simulink model "MicrogridControl"  (R2025b)
settings: Solver=VariableStepAuto  StartTime=0.0  StopTime=8  FixedStep=Ts  RelTol=1e-3
PreLoadFcn:
  | NormalOperation;
  | MicrogridControlParam;
undefined symbols (not defined in the file): base, bessModeInitial, bessSystem, bessVoltage, breakerStatus, DiscIntNeverNeededParam, ee_sli_rtmsupport, event, gcbh, generator, gflInverter, gfmInverter, Inertia, lineInductance, lineResistance, machine, plannedIsland, pmsm, powerLimit, powerQuality, PV, PVInverter, ref, resync, solar, solarInsolationChange, systemFrequency, Ts, windController, windSystem, windTurbine
libraries: nesl_utility x234, ee_lib x174, fl_lib x143, eeGeneralControl x137, simulink x78, eeTransforms x47, slpidlib x23, nesl_utility_internal x12, eePwmGenerator x9, eeSinusoidalMeasurementV2 x9, custom_lib x7, batteryecm_lib x6
(part 20 of 25)

== system MicrogridControl/BESS/BESS Integrated/Detailed/BESS Controller/Grid Forming/Power Control/ReactiveControl/Voltage  Reference Selection ==
  cntrlflag : Inport
  Qref : Inport  Port=2
  Qmeas : Inport  Port=3
  Vref : Inport  Port=4
  Vgdmeas : Inport  Port=5
  If : If
  If Action Subsystem : Subsystem  TreatAsAtomicUnit=on
  If Action Subsystem1 : Subsystem  TreatAsAtomicUnit=on
  Merge : Merge
  Rate Transition : RateTransition
  Vd : Outport
  wires:
  Rate Transition/1 -> If/1
  Vgdmeas/1 -> If Action Subsystem1/2(Vmeas)
  Vref/1 -> If Action Subsystem1/1(Vref)
  If Action Subsystem1/1(Voltage) -> Merge/2
  Qref/1 -> If Action Subsystem/1(Qref)
  Qmeas/1 -> If Action Subsystem/2(Qmeas)
  Merge/1 -> Vd/1
  cntrlflag/1 -> Rate Transition/1
  If/2 -> If Action Subsystem1/Action
  If Action Subsystem/1(Vd) -> Merge/1
  If/1 -> If Action Subsystem/Action

== system MicrogridControl/BESS/BESS Integrated/Detailed/BESS Controller/Grid Forming/VoltageCurrentControl/Controller/Id Current Limiting ==
  Imax : Inport
  Id : Inport  Port=2
  Abs : Abs  SaturateOnIntegerOverflow=off
  Switch : Switch  Criteria=u2 > Threshold  SaturateOnIntegerOverflow=off  InputSameDT=off
  Idref : Outport
  wires:
  Switch/1 -> Idref/1
  Imax/1 -> Switch/1, Abs/1
  Abs/1 -> Switch/2
  Id/1 -> Switch/3

== system MicrogridControl/BESS/BESS Integrated/Detailed/BESS Controller/Grid Forming/VoltageCurrentControl/Controller/Iq Current Limiting ==
  Imax : Inport
  Iq : Inport  Port=2
  Abs : Abs  SaturateOnIntegerOverflow=off
  Switch : Switch  Criteria=u2 > Threshold  SaturateOnIntegerOverflow=off  InputSameDT=off
  Iqref : Outport
  wires:
  Switch/1 -> Iqref/1
  Imax/1 -> Switch/1, Abs/1
  Abs/1 -> Switch/2
  Iq/1 -> Switch/3

== system MicrogridControl/BESS/BESS Integrated/Detailed/BESS Controller/Grid Forming/VoltageCurrentControl/Controller/Voltage control ==
  e : Inport
  resetBlackStart : Inport  Port=2
  Discrete-Time Integrator : DiscreteIntegrator  IntegratorMethod=Integration: Backward Euler  ExternalReset=level  SampleTime=voltControlTs  LimitOutput=on  UpperSaturationLimit=VdMaxCt  LowerSaturationLimit=VdMinCt  ICPrevOutput=DiscIntNeverNeededParam  ICPrevScaledInput=DiscIntNeverNeededParam
  Ki : Gain  Gain=VdIGain
  Kp : Gain  Gain=vdPGain
  Limit : Saturate  UpperLimit=VdMaxCt  LowerLimit=VdMinCt
  Scope : Scope  NumInputPorts=2
      settings: ActiveDisplayYMinimum=-2.29888  ActiveDisplayYMaximum=11.36654  DataLoggingVariableName=ScopeData7
  Scope1 : Scope
      settings: ActiveDisplayYMinimum=-0.22989  ActiveDisplayYMaximum=1.13665  DataLoggingVariableName=ScopeData8
  Sum7 : Sum  Inputs=|++
  u : Outport  VectorParamsAs1DForOutWhenUnconnected=off
  wires:
  resetBlackStart/1 -> Discrete-Time Integrator/2
  e/1 -> Scope1/1, Ki/1, Kp/1
  Sum7/1 -> Limit/1
  Ki/1 -> Discrete-Time Integrator/1
  Limit/1 -> u/1
  Kp/1 -> Scope/1, Sum7/1
  Discrete-Time Integrator/1 -> Scope/2, Sum7/2

== system MicrogridControl/BESS/BESS Integrated/Detailed/BESS Controller/Grid Forming/VoltageCurrentControl/Controller/Voltage control1 ==
  e : Inport
  resetBlackStart : Inport  Port=2
  Discrete-Time Integrator : DiscreteIntegrator  IntegratorMethod=Integration: Backward Euler  ExternalReset=level  SampleTime=voltControlTs  LimitOutput=on  UpperSaturationLimit=VqMaxCt  LowerSaturationLimit=VqMinCt  ICPrevOutput=DiscIntNeverNeededParam  ICPrevScaledInput=DiscIntNeverNeededParam
  Ki : Gain  Gain=VqIGain
  Kp : Gain  Gain=VqPGain
  Limit : Saturate  UpperLimit=VqMaxCt  LowerLimit=VqMinCt
  Sum7 : Sum  Inputs=|++
  u : Outport  VectorParamsAs1DForOutWhenUnconnected=off
  wires:
  resetBlackStart/1 -> Discrete-Time Integrator/2
  Limit/1 -> u/1
  Ki/1 -> Discrete-Time Integrator/1
  Kp/1 -> Sum7/1
  e/1 -> Kp/1, Ki/1
  Sum7/1 -> Limit/1
  Discrete-Time Integrator/1 -> Sum7/2

== system MicrogridControl/BESS/BESS Integrated/Detailed/BESS Controller/Grid Forming/VoltageCurrentControl/Controller/d-axis current control ==
  e : Inport
  resetBlackStart : Inport  Port=2
  Discrete-Time Integrator : DiscreteIntegrator  IntegratorMethod=Integration: Backward Euler  ExternalReset=level  SampleTime=currentControlTs  LimitOutput=on  UpperSaturationLimit=4  LowerSaturationLimit=-4  ICPrevOutput=DiscIntNeverNeededParam  ICPrevScaledInput=DiscIntNeverNeededParam
  Ki : Gain  Gain=IdIGain
  Kp : Gain  Gain=IdPGain
  Limit : Saturate  UpperLimit=4  LowerLimit=-4
  Sum7 : Sum  Inputs=|++
  u : Outport  VectorParamsAs1DForOutWhenUnconnected=off
  wires:
  resetBlackStart/1 -> Discrete-Time Integrator/2
  Ki/1 -> Discrete-Time Integrator/1
  Limit/1 -> u/1
  Kp/1 -> Sum7/1
  e/1 -> Kp/1, Ki/1
  Sum7/1 -> Limit/1
  Discrete-Time Integrator/1 -> Sum7/2

== system MicrogridControl/BESS/BESS Integrated/Detailed/BESS Controller/Grid Forming/VoltageCurrentControl/Controller/q-axis current control ==
  e : Inport
  resetBlackStart : Inport  Port=2
  Discrete-Time Integrator : DiscreteIntegrator  IntegratorMethod=Integration: Backward Euler  ExternalReset=level  SampleTime=currentControlTs  LimitOutput=on  UpperSaturationLimit=3  LowerSaturationLimit=-3  ICPrevOutput=DiscIntNeverNeededParam  ICPrevScaledInput=DiscIntNeverNeededParam
  Ki : Gain  Gain=IqIGain
  Kp : Gain  Gain=IqPGain
  Limit : Saturate  UpperLimit=3  LowerLimit=-3
  Sum7 : Sum  Inputs=|++
  u : Outport  VectorParamsAs1DForOutWhenUnconnected=off
  wires:
  resetBlackStart/1 -> Discrete-Time Integrator/2
  Discrete-Time Integrator/1 -> Sum7/2
  Limit/1 -> u/1
  Sum7/1 -> Limit/1
  e/1 -> Ki/1, Kp/1
  Kp/1 -> Sum7/1
  Ki/1 -> Discrete-Time Integrator/1

== system MicrogridControl/BESS/BESS Integrated1/Detailed/BESS Controller/Grid Forming/Current Limiting/CurrentLimitingMethod/currentLimitAndVirtual ==
  Igd : Inport
  Igq : Inport  Port=2
  Current Saturation : Subsystem
  CurrentLimitSelection : Stateflow chart  TreatAsAtomicUnit=on
  Math Function : Math  Operator=hypot
  Merge{,1..3} (4 alike) : Merge  Inputs=3
  No Fault Ride Through : Subsystem
  VI : Subsystem
  delVd : Outport
  delVq : Outport  Port=2
  Idmax : Outport  Port=3
  Iqmax : Outport  Port=4
  wires:
  [Imax] -> VI/3(Imax)
  [Imax] -> Current Saturation/3(Imaxsat)
  [noCtLt] -> No Fault Ride Through/Enable
  [satCtLt] -> Current Saturation/Enable
  [viCtLt] -> VI/Enable
  CurrentLimitSelection/4(satCurrentLimit) -> [satCtLt]
  CurrentLimitSelection/3(viCurrentLimit) -> [viCtLt]
  CurrentLimitSelection/2(noCurrentLimit) -> [noCtLt]
  CurrentLimitSelection/1(ismax) -> [Imax]
  Math Function/1 -> CurrentLimitSelection/1(Is)
  No Fault Ride Through/2(delVq) -> Merge1/3
  Merge3/1 -> Iqmax/1
  Current Saturation/2(delVq) -> Merge1/2
  No Fault Ride Through/4(iqmax) -> Merge3/3
  VI/3(idmax) -> Merge2/1
  VI/4(iqmax) -> Merge3/1
  Current Saturation/3(idmax) -> Merge2/2
  VI/2(delVq) -> Merge1/1
  Merge/1 -> delVd/1
  Current Saturation/4(iqmax) -> Merge3/2
  Current Saturation/1(delVd) -> Merge/2
  [Id] -> Math Function/1
  [Iq] -> Math Function/2
  VI/1(delVd) -> Merge/1
  No Fault Ride Through/3(idmax) -> Merge2/3
  No Fault Ride Through/1(delVd) -> Merge/3
  Igd/1 -> [Id], No Fault Ride Through/1(Id), Current Saturation/1(Id), VI/1(Id)
  Merge1/1 -> delVq/1
  Igq/1 -> [Iq], No Fault Ride Through/2(Iq), VI/2(Iq), Current Saturation/2(Iq)
  Merge2/1 -> Idmax/1

== system MicrogridControl/BESS/BESS Integrated1/Detailed/BESS Controller/Grid Forming/Current Limiting/CurrentLimitingMethod/currentSaturation ==
  note: Vs-delV
  Igd : Inport
  Igq : Inport  Port=2
  Compare : Subsystem
  Constant : Constant  Value=maxSatCurrentLimit
  Constant1 : Constant  Value=0
  Constant2 : Constant  Value=0
  If : If
  If Action Subsystem : Subsystem  TreatAsAtomicUnit=on
  If Action Subsystem1 : Subsystem  TreatAsAtomicUnit=on
  Math Function : Math  Operator=hypot
  Merge : Merge
  Merge1 : Merge
  Subtract : Sum  Inputs=+-
  delVd : Outport
  delVq : Outport  Port=2
  Idmax : Outport  Port=3
  Iqmax : Outport  Port=4
  wires:
  Merge1/1 -> Iqmax/1
  Merge/1 -> Idmax/1
  Constant1/1 -> delVd/1
  Constant2/1 -> delVq/1
  If Action Subsystem1/2(Iqmax) -> Merge1/2
  If Action Subsystem/2(Iqmax) -> Merge1/1
  If Action Subsystem1/1(Idmax) -> Merge/2
  If Action Subsystem/1(Idmax) -> Merge/1
  [Is] -> If Action Subsystem/1(Is)
  If/2 -> If Action Subsystem1/Action
  Compare/1(Out1) -> If/1
  Subtract/1 -> Compare/1(u)
  [Isq] -> If Action Subsystem/3(Isq)
  [Isd] -> If Action Subsystem/2(Isd)
  If/1 -> If Action Subsystem/Action
  Math Function/1 -> Subtract/2, [Is]  "Is"
  Constant/1 -> Subtract/1
  Igq/1 -> Math Function/2, [Isq]
  Igd/1 -> Math Function/1, [Isd]

== system MicrogridControl/BESS/BESS Integrated1/Detailed/BESS Controller/Grid Forming/Current Limiting/CurrentLimitingMethod/virtualImpedance ==
  note: Resistance coefficient
  note: X/R ratio
  Igd : Inport
  Igq : Inport  Port=2
  Constant : Constant  Value=maxVICurrentLimit
  Constant1 : Constant  Value=0
  Constant2 : Constant  Value=0
  Constant3 : Constant  Value=0
  Gain : Gain  Gain=ctLimitVirtualImp
  Gain1 : Gain  Gain=ctLimitXbyR
  Low-Pass Filter : eeGeneralControl/Low-Pass Filter (Discrete or Continuous)  K=1  T=currentVITimeConst  B=inf  A=-inf  init_option=Inherited from block input  x0=0  Ts=-1
  Math Function : Math  Operator=hypot
  Product{,1..3} (4 alike) : Product
  Relay : Relay  OnSwitchValue=0.01  OffSwitchValue=-0.05
  Saturation : Saturate  UpperLimit=1  LowerLimit=-1
  Saturation1 : Saturate  UpperLimit=1  LowerLimit=-1
  Sum : Sum  Inputs=|+-
  Sum1 : Sum  Inputs=|+-
  Sum2 : Sum  Inputs=++|
  Switch : Switch  Criteria=u2 > Threshold  SaturateOnIntegerOverflow=off  InputSameDT=off
  delVd : Outport
  delVq : Outport  Port=2
  Idmax : Outport  Port=3
  Iqmax : Outport  Port=4
  wires:
  Sum2/1 -> Saturation1/1
  Product3/1 -> Sum2/2
  Low-Pass Filter/1 -> Sum/1
  Saturation/1 -> delVd/1
  Relay/1 -> Switch/2
  Saturation1/1 -> delVq/1
  Igd/1 -> [Igd], Math Function/1
  Constant1/1 -> Switch/3
  Gain/1 -> Switch/1
  Constant3/1 -> Iqmax/1
  Constant2/1 -> Idmax/1
  [Igd] -> Product/2, Product1/1
  Switch/1 -> Product/1, Product3/2, Gain1/1
  [Igq] -> Product2/2, Product3/1
  Math Function/1 -> Low-Pass Filter/1  "Is"
  Constant/1 -> Sum/2  "IsMaxium"
  Product2/1 -> Sum1/2
  Product/1 -> Sum1/1
  Sum1/1 -> Saturation/1
  Gain1/1 -> Product2/1, Product1/2
  Product1/1 -> Sum2/1
  Igq/1 -> Math Function/2, [Igq]
  Sum/1 -> Relay/1, Gain/1

== system MicrogridControl/BESS/BESS Integrated1/Detailed/BESS Controller/Grid Forming/Grid Voltage Reactive Power Support/Modifying Active Power Reference/Computing New Active Power Ref ==
  Iq : Inport
  Vd : Inport  Port=2
  Abs : Abs  SaturateOnIntegerOverflow=off
  Constant : Constant  Value=maxVICurrentLimit*0.96
  Constant1 : Constant  Value=0
  Product : Product
  Sqrt : Sqrt
  Square : Math  Operator=square
  Square1 : Math  Operator=square
  Subtract : Sum  Inputs=-+
  Switch : Switch  Criteria=u2 > Threshold  Threshold=1.15  SaturateOnIntegerOverflow=off  InputSameDT=off
  Pref : Outport
  wires:
  Product/1 -> Pref/1
  Iq/1 -> Square/1
  Sqrt/1 -> Abs/1
  Vd/1 -> Product/1
  Constant1/1 -> Switch/1
  Square1/1 -> Subtract/2
  Square/1 -> Switch/2, Subtract/1
  Switch/1 -> Product/2
  Subtract/1 -> Sqrt/1
  Constant/1 -> Square1/1
  Abs/1 -> Switch/3

== system MicrogridControl/BESS/BESS Integrated1/Detailed/BESS Controller/Grid Forming/Grid Voltage Reactive Power Support/Modifying Reactive Power Reference/Changing the Power Reference ==
  Vs : Inport
  Vd : Inport  Port=2
  Pref : Inport  Port=3
  Qref : Inport  Port=4
  Enable : EnablePort
  ActivePowerReference : Subsystem
  Constant1 : Constant  Value=voltreference*0.96
  EstimateIdForGivenIq : Subsystem
  EstimateIqForReactivePower : Subsystem
  Max : MinMax  Function=max  Inputs=2
  ReactivePowerReference : Subsystem
  Prefv : Outport
  Qrefv : Outport  Port=2
  wires:
  Vd/1 -> EstimateIqForReactivePower/2(Vd)
  Qref/1 -> Max/2
  ReactivePowerReference/1(QrefNew) -> Max/1
  Pref/1 -> ActivePowerReference/3(Pref)
  EstimateIdForGivenIq/1(Id) -> ActivePowerReference/1(Id)
  Vs/1 -> ReactivePowerReference/1(Vd), EstimateIqForReactivePower/3(Vs), ActivePowerReference/2(Vd)
  Constant1/1 -> EstimateIqForReactivePower/1(Vmin)
  EstimateIqForReactivePower/1(Iq) -> ReactivePowerReference/2(Iq), EstimateIdForGivenIq/1(Iq)
  Max/1 -> Qrefv/1
  ActivePowerReference/1(PrefNew) -> Prefv/1

== system MicrogridControl/BESS/BESS Integrated1/Detailed/BESS Controller/Grid Forming/Grid Voltage Reactive Power Support/Modifying Reactive Power Reference/Hysteresis ==
  Vs : Inport
  AND : Logic  IconShape=distinctive  AllPortsSameDT=off  OutDataTypeStr=boolean
  Compare To Constant : simulink/Logic and Bit Operations/Compare To Constant  relop=<  const=0.9  OutDataTypeStr=boolean
  Compare To Constant1 : simulink/Logic and Bit Operations/Compare To Constant  relop=<  const=0.95  OutDataTypeStr=boolean
  D Latch : simulink_extras/Flip Flops/D Latch
  OR : Logic  Operator=OR  IconShape=distinctive  AllPortsSameDT=off  OutDataTypeStr=boolean
  Scope : Scope
      settings: ActiveDisplayYMinimum=0.96929  ActiveDisplayYMaximum=1.01111
  Terminator : Terminator
  LVFlag : Outport
  wires:
  Vs/1 -> Compare To Constant/1, Compare To Constant1/1, Scope/1
  Compare To Constant/1 -> OR/2, D Latch/2, D Latch/1
  D Latch/2 -> Terminator/1
  OR/1 -> LVFlag/1
  AND/1 -> OR/1
  D Latch/1 -> AND/2
  Compare To Constant1/1 -> AND/1

== system MicrogridControl/BESS/BESS Integrated1/Detailed/BESS Controller/Grid Forming/Grid Voltage Reactive Power Support/Modifying Reactive Power Reference/Not Altering the Power Reference ==
  Pref : Inport
  Qref : Inport  Port=2
  Enable : EnablePort
  Prefv : Outport
  Qrefv : Outport  Port=2
  wires:
  Qref/1 -> Qrefv/1
  Pref/1 -> Prefv/1

== system MicrogridControl/BESS/BESS Integrated1/Detailed/BESS Controller/Grid Forming/Measurement/Frequency Measurement/Frequency Measurement ==
  abc : Inport
  Constant : Constant
  Discrete-Time Integrator : DiscreteIntegrator  SampleTime=sampleTime  LimitOutput=on  ICPrevOutput=DiscIntNeverNeededParam  ICPrevScaledInput=DiscIntNeverNeededParam
  If : If  IfExpression=u1 > 0.9
  If Action Subsystem : Subsystem  TreatAsAtomicUnit=on
  If Action Subsystem1 : Subsystem  TreatAsAtomicUnit=on
  Merge : Merge
  Postive Sequence : Subsystem
  Freq : Outport
  wires:
  Postive Sequence/1(posSeq) -> If Action Subsystem/1(V)
  Merge/1 -> Freq/1
  If Action Subsystem1/1(Out1) -> Merge/2
  If Action Subsystem/1(Freq) -> Merge/1
  Constant/1 -> Discrete-Time Integrator/1
  abc/1 -> Postive Sequence/1(abc)
  Discrete-Time Integrator/1 -> If/1, If Action Subsystem/2(Time)
  If/2 -> If Action Subsystem1/Action
  If/1 -> If Action Subsystem/Action

== system MicrogridControl/BESS/BESS Integrated1/Detailed/BESS Controller/Grid Forming/Measurement/abc2dq/Supply Current to dq ==
  abc : Inport
  Angle : Inport  Port=2
  Demux : Demux  Outputs=3
  Park Transform : eeTransforms/Park Transform  AxisAlignment=D-axis  PowerInvariant=off
  Terminator : Terminator
  Igd : Outport  VectorParamsAs1DForOutWhenUnconnected=off
  Igq : Outport  Port=2  VectorParamsAs1DForOutWhenUnconnected=off
  wires:
  Angle/1 -> Park Transform/2
  abc/1 -> Park Transform/1
  Demux/1 -> Igd/1
  Demux/2 -> Igq/1
  Park Transform/1 -> Demux/1
  Demux/3 -> Terminator/1

== system MicrogridControl/BESS/BESS Integrated1/Detailed/BESS Controller/Grid Forming/Measurement/abc2dq/Supply Voltage  to dq1 ==
  Angle : Inport
  abc : Inport  Port=2
  Demux : Demux  Outputs=3
  Park Transform : eeTransforms/Park Transform  AxisAlignment=D-axis  PowerInvariant=off
  Terminator : Terminator
  Vgd : Outport  VectorParamsAs1DForOutWhenUnconnected=off
  Vgq : Outport  Port=2  VectorParamsAs1DForOutWhenUnconnected=off
  wires:
  Angle/1 -> Park Transform/2
  abc/1 -> Park Transform/1
  Demux/1 -> Vgd/1
  Demux/2 -> Vgq/1
  Park Transform/1 -> Demux/1
  Demux/3 -> Terminator/1

== system MicrogridControl/BESS/BESS Integrated1/Detailed/BESS Controller/Grid Forming/Power Control/ActivePowerControl/droopControl ==
  Pref : Inport
  Pmeas : Inport  Port=2
  fref : Inport  Port=3
  cntrlflag : Inport  Port=4
  fgrid : Inport  Port=5
  Add : Sum  Inputs=+-
  Constant : Constant
  Constant5 : Constant  Value=pi/2
  Gain : Gain  Gain=powerFreq*2*pi
  Integrator with Wrapped State (Discrete or Continuous) : eeGeneralControl/Integrator with Wrapped State (Discrete or Continuous)  LabelModeActiveChoice=Discrete  WrappedStateUpperValue=2*pi  WrappedStateLowerValue=0  x0=0  Ts=activePowerSampleTime
  Lead-Lag (Discrete or Continuous) : eeGeneralControl/Lead-Lag (Discrete or Continuous)  T1=droopT1  T2=droopT2  B=inf  A=-inf  init_option=Inherited from block input  x0=0  Ts=activePowerSampleTime
  Low-Pass Filter (Discrete or Continuous) : eeGeneralControl/Low-Pass Filter (Discrete or Continuous)  K=1  T=droopTC  B=inf  A=-inf  init_option=Specify as parameter  x0=0  Ts=activePowerSampleTime
  Scope : Scope
  Scope1 : Scope
  Scope2 : Scope
  Sum : Sum  Inputs=|-+
  Sum1 : Sum  Inputs=|-+
  Terminator : Terminator
  Terminator1 : Terminator
  Terminator2 : Terminator
  mp : Gain  Gain=droopSlope
  Theta : Outport
  w : Outport  Port=2
  wires:
  cntrlflag/1 -> Terminator2/1
  fref/1 -> Terminator1/1
  fgrid/1 -> Terminator/1
  Sum1/1 -> Gain/1
  Constant/1 -> Sum1/2
  Integrator with Wrapped State (Discrete or Continuous)/1 -> Add/1
  Lead-Lag (Discrete or Continuous)/1 -> Sum/2
  Gain/1 -> w/1, Integrator with Wrapped State (Discrete or Continuous)/1
  Pref/1 -> Sum/1
  Constant5/1 -> Add/2
  Add/1 -> Theta/1, Scope1/1
  Pmeas/1 -> Lead-Lag (Discrete or Continuous)/1
  Sum/1 -> mp/1, Scope/1
  mp/1 -> Low-Pass Filter (Discrete or Continuous)/1
  Low-Pass Filter (Discrete or Continuous)/1 -> Sum1/1, Scope2/1

== system MicrogridControl/BESS/BESS Integrated1/Detailed/BESS Controller/Grid Forming/Power Control/ActivePowerControl/vsmControl ==
  note: Damping power input
  note: Measured power
  Pref : Inport
  Pmeas : Inport  Port=2
  fref : Inport  Port=3
  cntrlflag : Inport  Port=4
  fgrid : Inport  Port=5
  Add : Sum  Inputs=+-
  Constant2 : Constant  Value=pi/2
  Damping Frequency : Subsystem  Variant=on  VariantControlMode=label  VariantControl=Choice  LabelModeActiveChoice=constFreq
  Discrete-Time Integrator : DiscreteIntegrator  IntegratorMethod=Integration: Backward Euler  InitialCondition=1  SampleTime=activePowerSampleTime  LimitOutput=on  UpperSaturationLimit=1.1  LowerSaturationLimit=0.9  ICPrevOutput=DiscIntNeverNeededParam  ICPrevScaledInput=DiscIntNeverNeededParam
  Gain : Gain  Gain=powerFreq*2*pi
  Gain1 : Gain  Gain=1/vsmInertiaTC
  Gain2 : Gain  Gain=vsmDampingConst*powerFreq
  Integrator with Wrapped State (Discrete or Continuous) : eeGeneralControl/Integrator with Wrapped State (Discrete or Continuous)  LabelModeActiveChoice=Discrete  WrappedStateUpperValue=2*pi  WrappedStateLowerValue=0  x0=0  Ts=activePowerSampleTime
  Low-Pass Filter (Discrete or Continuous) : eeGeneralControl/Low-Pass Filter (Discrete or Continuous)  K=1  T=vsmPmeasFilterTC  B=inf  A=-inf  init_option=Specify as parameter  x0=0  Ts=activePowerSampleTime
  Power Reference Selection : Subsystem
  Saturation : Saturate  UpperLimit=dampingPowerMaxLimit  LowerLimit=dampingPowerMinLimit
  Scope : Scope
  Sum1 : Sum  Inputs=-+-|
  Sum2 : Sum  Inputs=|+-
  Unit Delay : UnitDelay  SampleTime=-1  HasFrameUpgradeWarning=on
  Unit Delay1 : UnitDelay  SampleTime=-1  HasFrameUpgradeWarning=on
  Theta : Outport
  w : Outport  Port=2
  wires:
  [Wsm] -> Power Reference Selection/4(Wsm)
  Pmeas/1 -> Low-Pass Filter (Discrete or Continuous)/1
  fref/1 -> Power Reference Selection/3(fref)
  Pref/1 -> Power Reference Selection/2(Pref)
  cntrlflag/1 -> Power Reference Selection/1(cntrlflag)
  Damping Frequency/1(fmeas) -> Sum2/2
  fgrid/1 -> Damping Frequency/1(fref)
  Saturation/1 -> Sum1/3  "Pdamping"
  Unit Delay1/1 -> [Wsm]
  Unit Delay/1 -> Gain2/1
  Gain/1 -> w/1, Scope/1, Integrator with Wrapped State (Discrete or Continuous)/1
  Gain1/1 -> Discrete-Time Integrator/1
  Sum2/1 -> Unit Delay/1
  Power Reference Selection/1(power) -> Sum1/2
  Gain2/1 -> Saturation/1
  Low-Pass Filter (Discrete or Continuous)/1 -> Sum1/1
  Discrete-Time Integrator/1 -> Sum2/1, Unit Delay1/1, Gain/1
  Add/1 -> Theta/1
  Constant2/1 -> Add/2
  Sum1/1 -> Gain1/1  "Pinertia"
  Integrator with Wrapped State (Discrete or Continuous)/1 -> Add/1

== system MicrogridControl/BESS/BESS Integrated1/Detailed/BESS Controller/Grid Forming/Power Control/ReactiveControl/Voltage  Reference Selection ==
  cntrlflag : Inport
  Qref : Inport  Port=2
  Qmeas : Inport  Port=3
  Vref : Inport  Port=4
  Vgdmeas : Inport  Port=5
  If : If
  If Action Subsystem : Subsystem  TreatAsAtomicUnit=on
  If Action Subsystem1 : Subsystem  TreatAsAtomicUnit=on
  Merge : Merge
  Rate Transition : RateTransition
  Vd : Outport
  wires:
  Rate Transition/1 -> If/1
  Vgdmeas/1 -> If Action Subsystem1/2(Vmeas)
  Vref/1 -> If Action Subsystem1/1(Vref)
  If Action Subsystem1/1(Voltage) -> Merge/2
  Qref/1 -> If Action Subsystem/1(Qref)
  Qmeas/1 -> If Action Subsystem/2(Qmeas)
  Merge/1 -> Vd/1
  cntrlflag/1 -> Rate Transition/1
  If/2 -> If Action Subsystem1/Action
  If Action Subsystem/1(Vd) -> Merge/1
  If/1 -> If Action Subsystem/Action

== system MicrogridControl/BESS/BESS Integrated1/Detailed/BESS Controller/Grid Forming/VoltageCurrentControl/Controller/Id Current Limiting ==
  Imax : Inport
  Id : Inport  Port=2
  Abs : Abs  SaturateOnIntegerOverflow=off
  Switch : Switch  Criteria=u2 > Threshold  SaturateOnIntegerOverflow=off  InputSameDT=off
  Idref : Outport
  wires:
  Switch/1 -> Idref/1
  Imax/1 -> Switch/1, Abs/1
  Abs/1 -> Switch/2
  Id/1 -> Switch/3

== system MicrogridControl/BESS/BESS Integrated1/Detailed/BESS Controller/Grid Forming/VoltageCurrentControl/Controller/Iq Current Limiting ==
  Imax : Inport
  Iq : Inport  Port=2
  Abs : Abs  SaturateOnIntegerOverflow=off
  Switch : Switch  Criteria=u2 > Threshold  SaturateOnIntegerOverflow=off  InputSameDT=off
  Iqref : Outport
  wires:
  Switch/1 -> Iqref/1
  Imax/1 -> Switch/1, Abs/1
  Abs/1 -> Switch/2
  Iq/1 -> Switch/3

== system MicrogridControl/BESS/BESS Integrated1/Detailed/BESS Controller/Grid Forming/VoltageCurrentControl/Controller/Voltage control ==
  e : Inport
  resetBlackStart : Inport  Port=2
  Discrete-Time Integrator : DiscreteIntegrator  IntegratorMethod=Integration: Backward Euler  ExternalReset=level  SampleTime=voltControlTs  LimitOutput=on  UpperSaturationLimit=VdMaxCt  LowerSaturationLimit=VdMinCt  ICPrevOutput=DiscIntNeverNeededParam  ICPrevScaledInput=DiscIntNeverNeededParam
  Ki : Gain  Gain=VdIGain
  Kp : Gain  Gain=vdPGain
  Limit : Saturate  UpperLimit=VdMaxCt  LowerLimit=VdMinCt
  Scope : Scope  NumInputPorts=2
      settings: ActiveDisplayYMinimum=-2.29888  ActiveDisplayYMaximum=11.36654  DataLoggingVariableName=ScopeData7
  Scope1 : Scope
      settings: ActiveDisplayYMinimum=-0.22989  ActiveDisplayYMaximum=1.13665  DataLoggingVariableName=ScopeData8
  Sum7 : Sum  Inputs=|++
  u : Outport  VectorParamsAs1DForOutWhenUnconnected=off
  wires:
  resetBlackStart/1 -> Discrete-Time Integrator/2
  e/1 -> Scope1/1, Ki/1, Kp/1
  Sum7/1 -> Limit/1
  Ki/1 -> Discrete-Time Integrator/1
  Limit/1 -> u/1
  Kp/1 -> Scope/1, Sum7/1
  Discrete-Time Integrator/1 -> Scope/2, Sum7/2

== system MicrogridControl/BESS/BESS Integrated1/Detailed/BESS Controller/Grid Forming/VoltageCurrentControl/Controller/Voltage control1 ==
  e : Inport
  resetBlackStart : Inport  Port=2
  Discrete-Time Integrator : DiscreteIntegrator  IntegratorMethod=Integration: Backward Euler  ExternalReset=level  SampleTime=voltControlTs  LimitOutput=on  UpperSaturationLimit=VqMaxCt  LowerSaturationLimit=VqMinCt  ICPrevOutput=DiscIntNeverNeededParam  ICPrevScaledInput=DiscIntNeverNeededParam
  Ki : Gain  Gain=VqIGain
  Kp : Gain  Gain=VqPGain
  Limit : Saturate  UpperLimit=VqMaxCt  LowerLimit=VqMinCt
  Sum7 : Sum  Inputs=|++
  u : Outport  VectorParamsAs1DForOutWhenUnconnected=off
  wires:
  resetBlackStart/1 -> Discrete-Time Integrator/2
  Limit/1 -> u/1
  Ki/1 -> Discrete-Time Integrator/1
  Kp/1 -> Sum7/1
  e/1 -> Kp/1, Ki/1
  Sum7/1 -> Limit/1
  Discrete-Time Integrator/1 -> Sum7/2

== system MicrogridControl/BESS/BESS Integrated1/Detailed/BESS Controller/Grid Forming/VoltageCurrentControl/Controller/d-axis current control ==
  e : Inport
  resetBlackStart : Inport  Port=2
  Discrete-Time Integrator : DiscreteIntegrator  IntegratorMethod=Integration: Backward Euler  ExternalReset=level  SampleTime=currentControlTs  LimitOutput=on  UpperSaturationLimit=4  LowerSaturationLimit=-4  ICPrevOutput=DiscIntNeverNeededParam  ICPrevScaledInput=DiscIntNeverNeededParam
  Ki : Gain  Gain=IdIGain
  Kp : Gain  Gain=IdPGain
  Limit : Saturate  UpperLimit=4  LowerLimit=-4
  Sum7 : Sum  Inputs=|++
  u : Outport  VectorParamsAs1DForOutWhenUnconnected=off
  wires:
  resetBlackStart/1 -> Discrete-Time Integrator/2
  Ki/1 -> Discrete-Time Integrator/1
  Limit/1 -> u/1
  Kp/1 -> Sum7/1
  e/1 -> Kp/1, Ki/1
  Sum7/1 -> Limit/1
  Discrete-Time Integrator/1 -> Sum7/2

== system MicrogridControl/BESS/BESS Integrated1/Detailed/BESS Controller/Grid Forming/VoltageCurrentControl/Controller/q-axis current control ==
  e : Inport
  resetBlackStart : Inport  Port=2
  Discrete-Time Integrator : DiscreteIntegrator  IntegratorMethod=Integration: Backward Euler  ExternalReset=level  SampleTime=currentControlTs  LimitOutput=on  UpperSaturationLimit=3  LowerSaturationLimit=-3  ICPrevOutput=DiscIntNeverNeededParam  ICPrevScaledInput=DiscIntNeverNeededParam
  Ki : Gain  Gain=IqIGain
  Kp : Gain  Gain=IqPGain
  Limit : Saturate  UpperLimit=3  LowerLimit=-3
  Sum7 : Sum  Inputs=|++
  u : Outport  VectorParamsAs1DForOutWhenUnconnected=off
  wires:
  resetBlackStart/1 -> Discrete-Time Integrator/2
  Discrete-Time Integrator/1 -> Sum7/2
  Limit/1 -> u/1
  Sum7/1 -> Limit/1
  e/1 -> Ki/1, Kp/1
  Kp/1 -> Sum7/1
  Ki/1 -> Discrete-Time Integrator/1

== system MicrogridControl/BESS/BESS Integrated3/Detailed/BESS Controller/Grid Forming/Current Limiting/CurrentLimitingMethod/currentLimitAndVirtual ==
  Igd : Inport
  Igq : Inport  Port=2
  Current Saturation : Subsystem
  CurrentLimitSelection : Stateflow chart  TreatAsAtomicUnit=on
  Math Function : Math  Operator=hypot
  Merge{,1..3} (4 alike) : Merge  Inputs=3
  No Fault Ride Through : Subsystem
  VI : Subsystem
  delVd : Outport
  delVq : Outport  Port=2
  Idmax : Outport  Port=3
  Iqmax : Outport  Port=4
  wires:
  [Imax] -> VI/3(Imax)
  [Imax] -> Current Saturation/3(Imaxsat)
  [noCtLt] -> No Fault Ride Through/Enable
  [satCtLt] -> Current Saturation/Enable
  [viCtLt] -> VI/Enable
  CurrentLimitSelection/4(satCurrentLimit) -> [satCtLt]
  CurrentLimitSelection/3(viCurrentLimit) -> [viCtLt]
  CurrentLimitSelection/2(noCurrentLimit) -> [noCtLt]
  CurrentLimitSelection/1(ismax) -> [Imax]
  Math Function/1 -> CurrentLimitSelection/1(Is)
  No Fault Ride Through/2(delVq) -> Merge1/3
  Merge3/1 -> Iqmax/1
  Current Saturation/2(delVq) -> Merge1/2
  No Fault Ride Through/4(iqmax) -> Merge3/3
  VI/3(idmax) -> Merge2/1
  VI/4(iqmax) -> Merge3/1
  Current Saturation/3(idmax) -> Merge2/2
  VI/2(delVq) -> Merge1/1
  Merge/1 -> delVd/1
  Current Saturation/4(iqmax) -> Merge3/2
  Current Saturation/1(delVd) -> Merge/2
  [Id] -> Math Function/1
  [Iq] -> Math Function/2
  VI/1(delVd) -> Merge/1
  No Fault Ride Through/3(idmax) -> Merge2/3
  No Fault Ride Through/1(delVd) -> Merge/3
  Igd/1 -> [Id], No Fault Ride Through/1(Id), Current Saturation/1(Id), VI/1(Id)
  Merge1/1 -> delVq/1
  Igq/1 -> [Iq], No Fault Ride Through/2(Iq), VI/2(Iq), Current Saturation/2(Iq)
  Merge2/1 -> Idmax/1

== system MicrogridControl/BESS/BESS Integrated3/Detailed/BESS Controller/Grid Forming/Current Limiting/CurrentLimitingMethod/currentSaturation ==
  note: Vs-delV
  Igd : Inport
  Igq : Inport  Port=2
  Compare : Subsystem
  Constant : Constant  Value=maxSatCurrentLimit
  Constant1 : Constant  Value=0
  Constant2 : Constant  Value=0
  If : If
  If Action Subsystem : Subsystem  TreatAsAtomicUnit=on
  If Action Subsystem1 : Subsystem  TreatAsAtomicUnit=on
  Math Function : Math  Operator=hypot
  Merge : Merge
  Merge1 : Merge
  Subtract : Sum  Inputs=+-
  delVd : Outport
  delVq : Outport  Port=2
  Idmax : Outport  Port=3
  Iqmax : Outport  Port=4
  wires:
  Merge1/1 -> Iqmax/1
  Merge/1 -> Idmax/1
  Constant1/1 -> delVd/1
  Constant2/1 -> delVq/1
  If Action Subsystem1/2(Iqmax) -> Merge1/2
  If Action Subsystem/2(Iqmax) -> Merge1/1
  If Action Subsystem1/1(Idmax) -> Merge/2
  If Action Subsystem/1(Idmax) -> Merge/1
  [Is] -> If Action Subsystem/1(Is)
  If/2 -> If Action Subsystem1/Action
  Compare/1(Out1) -> If/1
  Subtract/1 -> Compare/1(u)
  [Isq] -> If Action Subsystem/3(Isq)
  [Isd] -> If Action Subsystem/2(Isd)
  If/1 -> If Action Subsystem/Action
  Math Function/1 -> Subtract/2, [Is]  "Is"
  Constant/1 -> Subtract/1
  Igq/1 -> Math Function/2, [Isq]
  Igd/1 -> Math Function/1, [Isd]

== system MicrogridControl/BESS/BESS Integrated3/Detailed/BESS Controller/Grid Forming/Current Limiting/CurrentLimitingMethod/virtualImpedance ==
  note: Resistance coefficient
  note: X/R ratio
  Igd : Inport
  Igq : Inport  Port=2
  Constant : Constant  Value=maxVICurrentLimit
  Constant1 : Constant  Value=0
  Constant2 : Constant  Value=0
  Constant3 : Constant  Value=0
  Gain : Gain  Gain=ctLimitVirtualImp
  Gain1 : Gain  Gain=ctLimitXbyR
  Low-Pass Filter : eeGeneralControl/Low-Pass Filter (Discrete or Continuous)  K=1  T=currentVITimeConst  B=inf  A=-inf  init_option=Inherited from block input  x0=0  Ts=-1
  Math Function : Math  Operator=hypot
  Product{,1..3} (4 alike) : Product
  Relay : Relay  OnSwitchValue=0.01  OffSwitchValue=-0.05
  Saturation : Saturate  UpperLimit=1  LowerLimit=-1
  Saturation1 : Saturate  UpperLimit=1  LowerLimit=-1
  Sum : Sum  Inputs=|+-
  Sum1 : Sum  Inputs=|+-
  Sum2 : Sum  Inputs=++|
  Switch : Switch  Criteria=u2 > Threshold  SaturateOnIntegerOverflow=off  InputSameDT=off
  delVd : Outport
  delVq : Outport  Port=2
  Idmax : Outport  Port=3
  Iqmax : Outport  Port=4
  wires:
  Sum2/1 -> Saturation1/1
  Product3/1 -> Sum2/2
  Low-Pass Filter/1 -> Sum/1
  Saturation/1 -> delVd/1
  Relay/1 -> Switch/2
  Saturation1/1 -> delVq/1
  Igd/1 -> [Igd], Math Function/1
  Constant1/1 -> Switch/3
  Gain/1 -> Switch/1
  Constant3/1 -> Iqmax/1
  Constant2/1 -> Idmax/1
  [Igd] -> Product/2, Product1/1
  Switch/1 -> Product/1, Product3/2, Gain1/1
  [Igq] -> Product2/2, Product3/1
  Math Function/1 -> Low-Pass Filter/1  "Is"
  Constant/1 -> Sum/2  "IsMaxium"
  Product2/1 -> Sum1/2
  Product/1 -> Sum1/1
  Sum1/1 -> Saturation/1
  Gain1/1 -> Product2/1, Product1/2
  Product1/1 -> Sum2/1
  Igq/1 -> Math Function/2, [Igq]
  Sum/1 -> Relay/1, Gain/1

== system MicrogridControl/BESS/BESS Integrated3/Detailed/BESS Controller/Grid Forming/Grid Voltage Reactive Power Support/Modifying Active Power Reference/Computing New Active Power Ref ==
  Iq : Inport
  Vd : Inport  Port=2
  Abs : Abs  SaturateOnIntegerOverflow=off
  Constant : Constant  Value=maxVICurrentLimit*0.96
  Constant1 : Constant  Value=0
  Product : Product
  Sqrt : Sqrt
  Square : Math  Operator=square
  Square1 : Math  Operator=square
  Subtract : Sum  Inputs=-+
  Switch : Switch  Criteria=u2 > Threshold  Threshold=1.15  SaturateOnIntegerOverflow=off  InputSameDT=off
  Pref : Outport
  wires:
  Product/1 -> Pref/1
  Iq/1 -> Square/1
  Sqrt/1 -> Abs/1
  Vd/1 -> Product/1
  Constant1/1 -> Switch/1
  Square1/1 -> Subtract/2
  Square/1 -> Switch/2, Subtract/1
  Switch/1 -> Product/2
  Subtract/1 -> Sqrt/1
  Constant/1 -> Square1/1
  Abs/1 -> Switch/3

== system MicrogridControl/BESS/BESS Integrated3/Detailed/BESS Controller/Grid Forming/Grid Voltage Reactive Power Support/Modifying Reactive Power Reference/Changing the Power Reference ==
  Vs : Inport
  Vd : Inport  Port=2
  Pref : Inport  Port=3
  Qref : Inport  Port=4
  Enable : EnablePort
  ActivePowerReference : Subsystem
  Constant1 : Constant  Value=voltreference*0.96
  EstimateIdForGivenIq : Subsystem
  EstimateIqForReactivePower : Subsystem
  Max : MinMax  Function=max  Inputs=2
  ReactivePowerReference : Subsystem
  Prefv : Outport
  Qrefv : Outport  Port=2
  wires:
  Vd/1 -> EstimateIqForReactivePower/2(Vd)
  Qref/1 -> Max/2
  ReactivePowerReference/1(QrefNew) -> Max/1
  Pref/1 -> ActivePowerReference/3(Pref)
  EstimateIdForGivenIq/1(Id) -> ActivePowerReference/1(Id)
  Vs/1 -> ReactivePowerReference/1(Vd), EstimateIqForReactivePower/3(Vs), ActivePowerReference/2(Vd)
  Constant1/1 -> EstimateIqForReactivePower/1(Vmin)
  EstimateIqForReactivePower/1(Iq) -> ReactivePowerReference/2(Iq), EstimateIdForGivenIq/1(Iq)
  Max/1 -> Qrefv/1
  ActivePowerReference/1(PrefNew) -> Prefv/1

== system MicrogridControl/BESS/BESS Integrated3/Detailed/BESS Controller/Grid Forming/Grid Voltage Reactive Power Support/Modifying Reactive Power Reference/Hysteresis ==
  Vs : Inport
  AND : Logic  IconShape=distinctive  AllPortsSameDT=off  OutDataTypeStr=boolean
  Compare To Constant : simulink/Logic and Bit Operations/Compare To Constant  relop=<  const=0.9  OutDataTypeStr=boolean
  Compare To Constant1 : simulink/Logic and Bit Operations/Compare To Constant  relop=<  const=0.95  OutDataTypeStr=boolean
  D Latch : simulink_extras/Flip Flops/D Latch
  OR : Logic  Operator=OR  IconShape=distinctive  AllPortsSameDT=off  OutDataTypeStr=boolean
  Scope : Scope
      settings: ActiveDisplayYMinimum=-1  ActiveDisplayYMaximum=1
  Terminator : Terminator
  LVFlag : Outport
  wires:
  Vs/1 -> Compare To Constant/1, Compare To Constant1/1, Scope/1
  Compare To Constant/1 -> OR/2, D Latch/2, D Latch/1
  D Latch/2 -> Terminator/1
  OR/1 -> LVFlag/1
  AND/1 -> OR/1
  D Latch/1 -> AND/2
  Compare To Constant1/1 -> AND/1

== system MicrogridControl/BESS/BESS Integrated3/Detailed/BESS Controller/Grid Forming/Grid Voltage Reactive Power Support/Modifying Reactive Power Reference/Not Altering the Power Reference ==
  Pref : Inport
  Qref : Inport  Port=2
  Enable : EnablePort
  Prefv : Outport
  Qrefv : Outport  Port=2
  wires:
  Qref/1 -> Qrefv/1
  Pref/1 -> Prefv/1

== system MicrogridControl/BESS/BESS Integrated3/Detailed/BESS Controller/Grid Forming/Measurement/Frequency Measurement/Frequency Measurement ==
  abc : Inport
  Constant : Constant
  Discrete-Time Integrator : DiscreteIntegrator  SampleTime=sampleTime  LimitOutput=on  ICPrevOutput=DiscIntNeverNeededParam  ICPrevScaledInput=DiscIntNeverNeededParam
  If : If  IfExpression=u1 > 0.9
  If Action Subsystem : Subsystem  TreatAsAtomicUnit=on
  If Action Subsystem1 : Subsystem  TreatAsAtomicUnit=on
  Merge : Merge
  Postive Sequence : Subsystem
  Freq : Outport
  wires:
  Postive Sequence/1(posSeq) -> If Action Subsystem/1(V)
  Merge/1 -> Freq/1
  If Action Subsystem1/1(Out1) -> Merge/2
  If Action Subsystem/1(Freq) -> Merge/1
  Constant/1 -> Discrete-Time Integrator/1
  abc/1 -> Postive Sequence/1(abc)
  Discrete-Time Integrator/1 -> If/1, If Action Subsystem/2(Time)
  If/2 -> If Action Subsystem1/Action
  If/1 -> If Action Subsystem/Action

== system MicrogridControl/BESS/BESS Integrated3/Detailed/BESS Controller/Grid Forming/Measurement/abc2dq/Supply Current to dq ==
  abc : Inport
  Angle : Inport  Port=2
  Demux : Demux  Outputs=3
  Park Transform : eeTransforms/Park Transform  AxisAlignment=D-axis  PowerInvariant=off
  Terminator : Terminator
  Igd : Outport  VectorParamsAs1DForOutWhenUnconnected=off
  Igq : Outport  Port=2  VectorParamsAs1DForOutWhenUnconnected=off
  wires:
  Angle/1 -> Park Transform/2
  abc/1 -> Park Transform/1
  Demux/1 -> Igd/1
  Demux/2 -> Igq/1
  Park Transform/1 -> Demux/1
  Demux/3 -> Terminator/1

== system MicrogridControl/BESS/BESS Integrated3/Detailed/BESS Controller/Grid Forming/Measurement/abc2dq/Supply Voltage  to dq1 ==
  Angle : Inport
  abc : Inport  Port=2
  Demux : Demux  Outputs=3
  Park Transform : eeTransforms/Park Transform  AxisAlignment=D-axis  PowerInvariant=off
  Terminator : Terminator
  Vgd : Outport  VectorParamsAs1DForOutWhenUnconnected=off
  Vgq : Outport  Port=2  VectorParamsAs1DForOutWhenUnconnected=off
  wires:
  Angle/1 -> Park Transform/2
  abc/1 -> Park Transform/1
  Demux/1 -> Vgd/1
  Demux/2 -> Vgq/1
  Park Transform/1 -> Demux/1
  Demux/3 -> Terminator/1

== system MicrogridControl/BESS/BESS Integrated3/Detailed/BESS Controller/Grid Forming/Power Control/ActivePowerControl/droopControl ==
  Pref : Inport
  Pmeas : Inport  Port=2
  fref : Inport  Port=3
  cntrlflag : Inport  Port=4
  fgrid : Inport  Port=5
  Add : Sum  Inputs=+-
  Constant : Constant
  Constant5 : Constant  Value=pi/2
  Gain : Gain  Gain=powerFreq*2*pi
  Integrator with Wrapped State (Discrete or Continuous) : eeGeneralControl/Integrator with Wrapped State (Discrete or Continuous)  LabelModeActiveChoice=Discrete  WrappedStateUpperValue=2*pi  WrappedStateLowerValue=0  x0=0  Ts=activePowerSampleTime
  Lead-Lag (Discrete or Continuous) : eeGeneralControl/Lead-Lag (Discrete or Continuous)  T1=droopT1  T2=droopT2  B=inf  A=-inf  init_option=Inherited from block input  x0=0  Ts=activePowerSampleTime
  Low-Pass Filter (Discrete or Continuous) : eeGeneralControl/Low-Pass Filter (Discrete or Continuous)  K=1  T=droopTC  B=inf  A=-inf  init_option=Specify as parameter  x0=0  Ts=activePowerSampleTime
  Scope : Scope
      settings: ActiveDisplayYMinimum=-1  ActiveDisplayYMaximum=1
  Scope1 : Scope
      settings: ActiveDisplayYMinimum=-2.356194275632717  ActiveDisplayYMaximum=5.4977852127454865
  Scope2 : Scope
      settings: ActiveDisplayYMinimum=-3.8720774562233728  ActiveDisplayYMaximum=1.5560107506901362
  Sum : Sum  Inputs=|-+
  Sum1 : Sum  Inputs=|-+
  Terminator : Terminator
  Terminator1 : Terminator
  Terminator2 : Terminator
  mp : Gain  Gain=droopSlope
  Theta : Outport
  w : Outport  Port=2
  wires:
  cntrlflag/1 -> Terminator2/1
  fref/1 -> Terminator1/1
  fgrid/1 -> Terminator/1
  Sum1/1 -> Gain/1
  Constant/1 -> Sum1/2
  Integrator with Wrapped State (Discrete or Continuous)/1 -> Add/1
  Lead-Lag (Discrete or Continuous)/1 -> Sum/2
  Gain/1 -> w/1, Integrator with Wrapped State (Discrete or Continuous)/1
  Pref/1 -> Sum/1
  Constant5/1 -> Add/2
  Add/1 -> Theta/1, Scope1/1
  Pmeas/1 -> Lead-Lag (Discrete or Continuous)/1
  Sum/1 -> mp/1, Scope/1
  mp/1 -> Low-Pass Filter (Discrete or Continuous)/1
  Low-Pass Filter (Discrete or Continuous)/1 -> Sum1/1, Scope2/1

== system MicrogridControl/BESS/BESS Integrated3/Detailed/BESS Controller/Grid Forming/Power Control/ActivePowerControl/vsmControl ==
  note: Damping power input
  note: Measured power
  Pref : Inport
  Pmeas : Inport  Port=2
  fref : Inport  Port=3
  cntrlflag : Inport  Port=4
  fgrid : Inport  Port=5
  Add : Sum  Inputs=+-
  Constant2 : Constant  Value=pi/2
  Damping Frequency : Subsystem  Variant=on  VariantControlMode=label  VariantControl=Choice  LabelModeActiveChoice=constFreq
  Discrete-Time Integrator : DiscreteIntegrator  IntegratorMethod=Integration: Backward Euler  InitialCondition=1  SampleTime=activePowerSampleTime  LimitOutput=on  UpperSaturationLimit=1.1  LowerSaturationLimit=0.9  ICPrevOutput=DiscIntNeverNeededParam  ICPrevScaledInput=DiscIntNeverNeededParam
  Gain : Gain  Gain=powerFreq*2*pi
  Gain1 : Gain  Gain=1/vsmInertiaTC
  Gain2 : Gain  Gain=vsmDampingConst*powerFreq
  Integrator with Wrapped State (Discrete or Continuous) : eeGeneralControl/Integrator with Wrapped State (Discrete or Continuous)  LabelModeActiveChoice=Discrete  WrappedStateUpperValue=2*pi  WrappedStateLowerValue=0  x0=0  Ts=activePowerSampleTime
  Low-Pass Filter (Discrete or Continuous) : eeGeneralControl/Low-Pass Filter (Discrete or Continuous)  K=1  T=vsmPmeasFilterTC  B=inf  A=-inf  init_option=Specify as parameter  x0=0  Ts=activePowerSampleTime
  Power Reference Selection : Subsystem
  Saturation : Saturate  UpperLimit=dampingPowerMaxLimit  LowerLimit=dampingPowerMinLimit
  Scope : Scope
      settings: ActiveDisplayYMinimum=-1  ActiveDisplayYMaximum=1
  Scope1 : Scope  NumInputPorts=3
      settings: ActiveDisplayYMinimum=-0.23047094467192353  ActiveDisplayYMaximum=1.365795688880348  DataLoggingVariableName=ScopeData48
  Scope2 : Scope  NumInputPorts=2
      settings: ActiveDisplayYMinimum=-1  ActiveDisplayYMaximum=1  DataLoggingVariableName=ScopeData49
  Sum1 : Sum  Inputs=-+-|
  Sum2 : Sum  Inputs=|+-
  Unit Delay : UnitDelay  SampleTime=-1  HasFrameUpgradeWarning=on
  Unit Delay1 : UnitDelay  SampleTime=-1  HasFrameUpgradeWarning=on
  Theta : Outport
  w : Outport  Port=2
  wires:
  [Wsm] -> Power Reference Selection/4(Wsm)
  Pmeas/1 -> Low-Pass Filter (Discrete or Continuous)/1
  fref/1 -> Power Reference Selection/3(fref)
  Pref/1 -> Power Reference Selection/2(Pref)
  cntrlflag/1 -> Power Reference Selection/1(cntrlflag)
  Damping Frequency/1(fmeas) -> Sum2/2
  fgrid/1 -> Damping Frequency/1(fref)
  Saturation/1 -> Scope1/3, Sum1/3  "Pdamping"
  Unit Delay1/1 -> [Wsm]
  Unit Delay/1 -> Gain2/1
  Gain/1 -> w/1, Scope/1, Integrator with Wrapped State (Discrete or Continuous)/1
  Gain1/1 -> Scope2/1, Discrete-Time Integrator/1
  Sum2/1 -> Unit Delay/1
  Power Reference Selection/1(power) -> Scope1/2, Sum1/2
  Gain2/1 -> Saturation/1
  Low-Pass Filter (Discrete or Continuous)/1 -> Sum1/1, Scope1/1
  Discrete-Time Integrator/1 -> Sum2/1, Unit Delay1/1, Scope2/2, Gain/1
  Add/1 -> Theta/1
  Constant2/1 -> Add/2
  Sum1/1 -> Gain1/1  "Pinertia"
  Integrator with Wrapped State (Discrete or Continuous)/1 -> Add/1

== system MicrogridControl/BESS/BESS Integrated3/Detailed/BESS Controller/Grid Forming/Power Control/ReactiveControl/Voltage  Reference Selection ==
  cntrlflag : Inport
  Qref : Inport  Port=2
  Qmeas : Inport  Port=3
  Vref : Inport  Port=4
  Vgdmeas : Inport  Port=5
  If : If
  If Action Subsystem : Subsystem  TreatAsAtomicUnit=on
  If Action Subsystem1 : Subsystem  TreatAsAtomicUnit=on
  Merge : Merge
  Rate Transition : RateTransition
  Vd : Outport
  wires:
  Rate Transition/1 -> If/1
  Vgdmeas/1 -> If Action Subsystem1/2(Vmeas)
  Vref/1 -> If Action Subsystem1/1(Vref)
  If Action Subsystem1/1(Voltage) -> Merge/2
  Qref/1 -> If Action Subsystem/1(Qref)
  Qmeas/1 -> If Action Subsystem/2(Qmeas)
  Merge/1 -> Vd/1
  cntrlflag/1 -> Rate Transition/1
  If/2 -> If Action Subsystem1/Action
  If Action Subsystem/1(Vd) -> Merge/1
  If/1 -> If Action Subsystem/Action

== system MicrogridControl/BESS/BESS Integrated3/Detailed/BESS Controller/Grid Forming/VoltageCurrentControl/Controller/Id Current Limiting ==
  Imax : Inport
  Id : Inport  Port=2
  Abs : Abs  SaturateOnIntegerOverflow=off
  Switch : Switch  Criteria=u2 > Threshold  SaturateOnIntegerOverflow=off  InputSameDT=off
  Idref : Outport
  wires:
  Switch/1 -> Idref/1
  Imax/1 -> Switch/1, Abs/1
  Abs/1 -> Switch/2
  Id/1 -> Switch/3

== system MicrogridControl/BESS/BESS Integrated3/Detailed/BESS Controller/Grid Forming/VoltageCurrentControl/Controller/Iq Current Limiting ==
  Imax : Inport
  Iq : Inport  Port=2
  Abs : Abs  SaturateOnIntegerOverflow=off
  Switch : Switch  Criteria=u2 > Threshold  SaturateOnIntegerOverflow=off  InputSameDT=off
  Iqref : Outport
  wires:
  Switch/1 -> Iqref/1
  Imax/1 -> Switch/1, Abs/1
  Abs/1 -> Switch/2
  Iq/1 -> Switch/3

== system MicrogridControl/BESS/BESS Integrated3/Detailed/BESS Controller/Grid Forming/VoltageCurrentControl/Controller/Voltage control ==
  e : Inport
  resetBlackStart : Inport  Port=2
  Discrete-Time Integrator : DiscreteIntegrator  IntegratorMethod=Integration: Backward Euler  ExternalReset=level  SampleTime=voltControlTs  LimitOutput=on  UpperSaturationLimit=VdMaxCt  LowerSaturationLimit=VdMinCt  ICPrevOutput=DiscIntNeverNeededParam  ICPrevScaledInput=DiscIntNeverNeededParam
  Ki : Gain  Gain=VdIGain
  Kp : Gain  Gain=vdPGain
  Limit : Saturate  UpperLimit=VdMaxCt  LowerLimit=VdMinCt
  Scope : Scope  NumInputPorts=2
      settings: ActiveDisplayYMinimum=-2.29888  ActiveDisplayYMaximum=11.36654  DataLoggingVariableName=ScopeData7
  Scope1 : Scope
      settings: ActiveDisplayYMinimum=-0.22989  ActiveDisplayYMaximum=1.13665  DataLoggingVariableName=ScopeData8
  Sum7 : Sum  Inputs=|++
  u : Outport  VectorParamsAs1DForOutWhenUnconnected=off
  wires:
  resetBlackStart/1 -> Discrete-Time Integrator/2
  e/1 -> Scope1/1, Ki/1, Kp/1
  Sum7/1 -> Limit/1
  Ki/1 -> Discrete-Time Integrator/1
  Limit/1 -> u/1
  Kp/1 -> Scope/1, Sum7/1
  Discrete-Time Integrator/1 -> Scope/2, Sum7/2

== system MicrogridControl/BESS/BESS Integrated3/Detailed/BESS Controller/Grid Forming/VoltageCurrentControl/Controller/Voltage control1 ==
  e : Inport
  resetBlackStart : Inport  Port=2
  Discrete-Time Integrator : DiscreteIntegrator  IntegratorMethod=Integration: Backward Euler  ExternalReset=level  SampleTime=voltControlTs  LimitOutput=on  UpperSaturationLimit=VqMaxCt  LowerSaturationLimit=VqMinCt  ICPrevOutput=DiscIntNeverNeededParam  ICPrevScaledInput=DiscIntNeverNeededParam
  Ki : Gain  Gain=VqIGain
  Kp : Gain  Gain=VqPGain
  Limit : Saturate  UpperLimit=VqMaxCt  LowerLimit=VqMinCt
  Sum7 : Sum  Inputs=|++
  u : Outport  VectorParamsAs1DForOutWhenUnconnected=off
  wires:
  resetBlackStart/1 -> Discrete-Time Integrator/2
  Limit/1 -> u/1
  Ki/1 -> Discrete-Time Integrator/1
  Kp/1 -> Sum7/1
  e/1 -> Kp/1, Ki/1
  Sum7/1 -> Limit/1
  Discrete-Time Integrator/1 -> Sum7/2

== system MicrogridControl/BESS/BESS Integrated3/Detailed/BESS Controller/Grid Forming/VoltageCurrentControl/Controller/d-axis current control ==
  e : Inport
  resetBlackStart : Inport  Port=2
  Discrete-Time Integrator : DiscreteIntegrator  IntegratorMethod=Integration: Backward Euler  ExternalReset=level  SampleTime=currentControlTs  LimitOutput=on  UpperSaturationLimit=4  LowerSaturationLimit=-4  ICPrevOutput=DiscIntNeverNeededParam  ICPrevScaledInput=DiscIntNeverNeededParam
  Ki : Gain  Gain=IdIGain
  Kp : Gain  Gain=IdPGain
  Limit : Saturate  UpperLimit=4  LowerLimit=-4
  Sum7 : Sum  Inputs=|++
  u : Outport  VectorParamsAs1DForOutWhenUnconnected=off
  wires:
  resetBlackStart/1 -> Discrete-Time Integrator/2
  Ki/1 -> Discrete-Time Integrator/1
  Limit/1 -> u/1
  Kp/1 -> Sum7/1
  e/1 -> Kp/1, Ki/1
  Sum7/1 -> Limit/1
  Discrete-Time Integrator/1 -> Sum7/2

== system MicrogridControl/BESS/BESS Integrated3/Detailed/BESS Controller/Grid Forming/VoltageCurrentControl/Controller/q-axis current control ==
  e : Inport
  resetBlackStart : Inport  Port=2
  Discrete-Time Integrator : DiscreteIntegrator  IntegratorMethod=Integration: Backward Euler  ExternalReset=level  SampleTime=currentControlTs  LimitOutput=on  UpperSaturationLimit=3  LowerSaturationLimit=-3  ICPrevOutput=DiscIntNeverNeededParam  ICPrevScaledInput=DiscIntNeverNeededParam
  Ki : Gain  Gain=IqIGain
  Kp : Gain  Gain=IqPGain
  Limit : Saturate  UpperLimit=3  LowerLimit=-3
  Sum7 : Sum  Inputs=|++
  u : Outport  VectorParamsAs1DForOutWhenUnconnected=off
  wires:
  resetBlackStart/1 -> Discrete-Time Integrator/2
  Discrete-Time Integrator/1 -> Sum7/2
  Limit/1 -> u/1
  Sum7/1 -> Limit/1
  e/1 -> Ki/1, Kp/1
  Kp/1 -> Sum7/1
  Ki/1 -> Discrete-Time Integrator/1
